simulink model "model_zlin"  (R2017a)
settings: Solver=ode15s  StartTime=0.0  StopTime=10  FixedStep=1e-3  MaxStep=1e-3  RelTol=1e-3
values from neighbouring files (symbols this model uses):
  dq = 1    [model.m]
  k = ((n+1)*gs*cs*Tp-(n+1)*gs*cs*Tpracy)/((n+1)*qpracy*gs*cs+m*v*c)    (= 11.036036036)    [model.m]
  Tczas = M*c/((n+1)*qpracy*gs*cs+m*v*c)    (= 1.57657657658)    [model.m]
  Tpracy = 800    [model.m]    (also in stat.m = (A*Tp*qpracy+B*T0)./(A*qpracy+B))
settings Model: Creator=Piotr  LastModifiedBy=Piotr

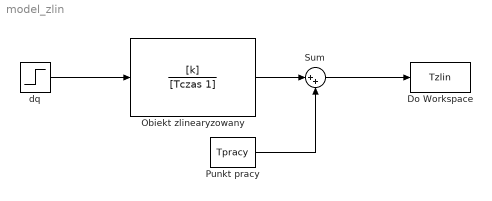
== system model_zlin ==
  Do Workspace : ToWorkspace  VariableName=Tzlin  SaveFormat=Timeseries  SampleTime=1e-3
  Obiekt zlinearyzowany : TransferFcn  Numerator=[k]  Denominator=[Tczas 1]
  Punkt pracy : Constant  Value=Tpracy
  Sum : Sum  Inputs=|++
  dq : Step  Time=0  After=dq  SampleTime=0
  wires:
  dq/1 -> Obiekt zlinearyzowany/1
  Obiekt zlinearyzowany/1 -> Sum/1
  Punkt pracy/1 -> Sum/2
  Sum/1 -> Do Workspace/1
